simulink model "dc_scenario_3"  (R2016a)
settings: Solver=FixedStepAuto  StartTime=0.0  StopTime=30.0  RelTol=1e-3
undefined symbols (not defined in the file or in its folder): DiscIntNeverNeededParam, sigbuilder_block
libraries: cstblocks x2, simulink x1, fuzblock x1
settings Model: Creator=Admin  LastModifiedBy=Admin

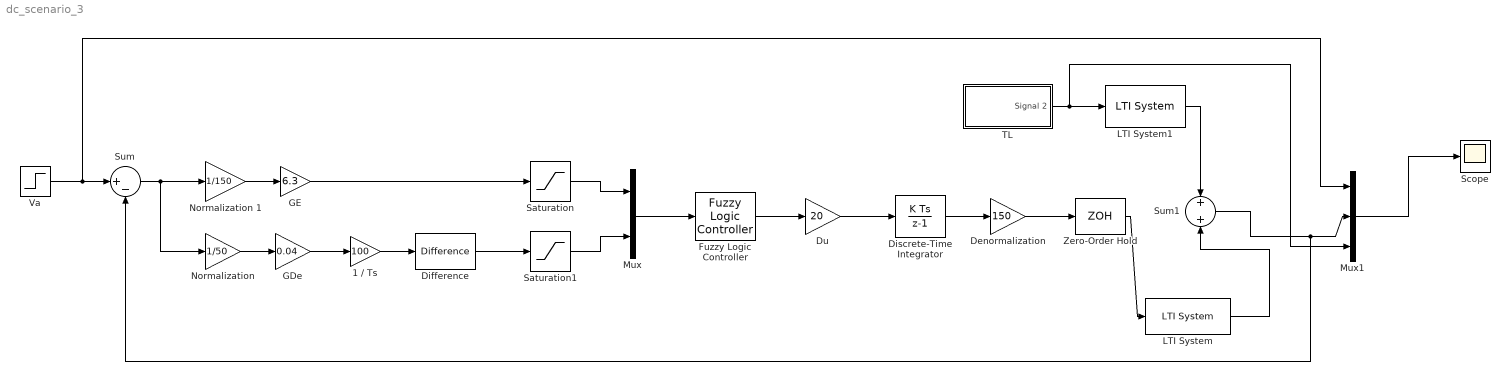
== system dc_scenario_3 ==
  1 / Ts : Gain  Gain=100
  Denormalization : Gain  Gain=150
  Difference : simulink/Discrete/Difference  ICPrevInput=0.0  OutMin=[]  OutMax=[]  OutDataType=fixdt(1, 16)  OutScaling=2^-10  DoSatur=off
  Discrete-Time Integrator : DiscreteIntegrator  InitialConditionSetting=State (most efficient)  SampleTime=0.01  ICPrevOutput=DiscIntNeverNeededParam  ICPrevScaledInput=DiscIntNeverNeededParam
  Du : Gain  Gain=20
  Fuzzy Logic Controller : fuzblock/Fuzzy Logic  Controller  fis=['model.fis']
  GDe : Gain  Gain=0.04
  GE : Gain  Gain=6.3
  LTI System : cstblocks/LTI System  sys=tf(18.69,[1 12.064])  IC=[]
  LTI System1 : cstblocks/LTI System  sys=tf([-2.92 -2.92*440],[1 12.064])  IC=[]
  Mux : Mux  Inputs=2
  Mux1 : Mux  Inputs=3
  Normalization : Gain  Gain=1/50
  Normalization 1 : Gain  Gain=1/150
  Saturation : Saturate  UpperLimit=1  LowerLimit=-1
  Saturation1 : Saturate  UpperLimit=1  LowerLimit=-1
  Scope : Scope
  Sum : Sum  Inputs=|+-
  Sum1 : Sum  Inputs=+|+
  TL : Subsystem  Tag=STV Subsys  LoadFcn=sigbuilder_block('load');  StartFcn=sigbuilder_block('start');  StopFcn=sigbuilder_block('stop');  ClipboardFcn=sigbuilder_block('clipboard');  mask(Sigbuilder block){}
      mask help: Simulink:masks:SigbuilderBlock_MD
      mask init:
      | if ~strcmp(get_param(bdroot(gcbh),'SimulationStatus'),'stopped') tuvar = sigbuilder_block('maskInit'); end
      settings: CopyFcn=sigbuilder_block('copy');  DeleteFcn=sigbuilder_block('delete');  ModelCloseFcn=sigbuilder_block('modelClose');  PreSaveFcn=sigbuilder_block('preSave');  PauseFcn=sigbuilder_block('pause');  ContinueFcn=sigbuilder_block('continue');  NameChangeFcn=sigbuilder_block('namechange');  OpenFcn=sigbuilder_block('open',[437.25 153 550.5 359.25 ]);  CloseFcn=sigbuilder_block('close');
      mask Display: plot(0, 0, 100, 100,[2, 2, 32, 32, 2], [68, 8, 8, 68, 68],[32, 2], [38, 38], [32, 19, 2],[53, 60, 44], [32, 17, 17, 2],[16, 16, 31, 31]);txt = getActiveGroup(gcbh);text(2, 100, txt,'verticalAlignment', 'top');
  Va : Step  Time=0  After=150  SampleTime=0.01
  Zero-Order Hold : ZeroOrderHold  SampleTime=0.01
  wires:
  Sum/1 -> Normalization/1, Normalization 1/1
  Normalization 1/1 -> GE/1
  Normalization/1 -> GDe/1
  GDe/1 -> 1 / Ts/1
  1 / Ts/1 -> Difference/1
  Difference/1 -> Saturation1/1
  GE/1 -> Saturation/1
  Saturation/1 -> Mux/1
  Saturation1/1 -> Mux/2
  Mux/1 -> Fuzzy Logic Controller/1
  Fuzzy Logic Controller/1 -> Du/1
  Du/1 -> Discrete-Time Integrator/1
  Discrete-Time Integrator/1 -> Denormalization/1
  Denormalization/1 -> Zero-Order Hold/1
  Zero-Order Hold/1 -> LTI System/1
  Mux1/1 -> Scope/1
  Va/1 -> Mux1/1, Sum/1
  LTI System1/1 -> Sum1/1
  LTI System/1 -> Sum1/2
  Sum1/1 -> Sum/2, Mux1/2
  TL/1(Signal 2) -> Mux1/3, LTI System1/1

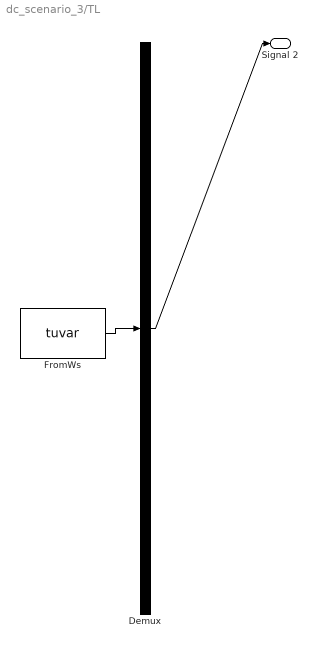
== system dc_scenario_3/TL ==
  Demux : Demux  Tag=STV Demux  Outputs=1
  FromWs : FromWorkspace  Tag=STV FromWs  VariableName=tuvar  SampleTime=0
      SigBuilderData=|
      | common.afterFinalStr = 'Extrapolate'
      | common.sampleTime = 0
      | dataSet.timeRange = [0 30]
      | dataSet.name = 'Group 1'
      | sbobj.Groups.Name = 'Group 1'
      | sbobj.Groups.Signals.Name = 'Signal 2'
      | sbobj.Groups.Signals.XData = [0 10 10 20 20 30]
      | sbobj.Groups.Signals.YData = [0 0 1 1 0 0]
      | sbobj.Groups.TimeRange = [0 30]
  Signal 2 : Outport  Tag=STV Outport
  wires:
  FromWs/1 -> Demux/1
  Demux/1 -> Signal 2/1
